simulink model "thermalBuilding3000"  (Simulink 8.3)
settings: Solver=ode5  StartTime=0.0  StopTime=24  FixedStep=stepSize  RelTol=1e-3
model workspace: external: MAT-File C:\Users\salanda\Desktop\Smart-Building/Data/wsVars/thermalBuilding3000WS.mat (data not in the file)
undefined symbols (not defined in the file): Ca, Ceq, cost, Mafc, Mafh, Req, Rwall, TAout, TCooler, THeater, TInit, TSet1, TSet2, TSet3
(part 2 of 2)

== system thermalBuilding3000/Building/Room2/Controller2/Reference Temperature/F2C   converter1 ==
  F : Inport
  Constant : Constant  Value=32  OutDataTypeStr=Inherit: Inherit via back propagation
  Gain1 : Gain  Gain=5/9  SaturateOnIntegerOverflow=on  OutDataTypeStr=Inherit: Same as input  ParamDataTypeStr=Inherit: Same as input
  Sum : Sum  Inputs=+-  SaturateOnIntegerOverflow=on  InputSameDT=on  OutDataTypeStr=Inherit: Same as first input
  C : Outport
  wires:
  Constant/1 -> Sum/2
  Gain1/1 -> C/1
  Sum/1 -> Gain1/1
  F/1 -> Sum/1

== system thermalBuilding3000/Building/Room3/Controller3/Reference Temperature/F2C   converter1 ==
  F : Inport
  Constant : Constant  Value=32  OutDataTypeStr=Inherit: Inherit via back propagation
  Gain1 : Gain  Gain=5/9  SaturateOnIntegerOverflow=on  OutDataTypeStr=Inherit: Same as input  ParamDataTypeStr=Inherit: Same as input
  Sum : Sum  Inputs=+-  SaturateOnIntegerOverflow=on  InputSameDT=on  OutDataTypeStr=Inherit: Same as first input
  C : Outport
  wires:
  Constant/1 -> Sum/2
  Gain1/1 -> C/1
  Sum/1 -> Gain1/1
  F/1 -> Sum/1
